simulink model "MyRhoVar"  (Simulink 7.9)
settings: Solver=FixedStepDiscrete  StartTime=0.0  StopTime=1e8  FixedStep=1  RelTol=1e-3
(part 2 of 3)

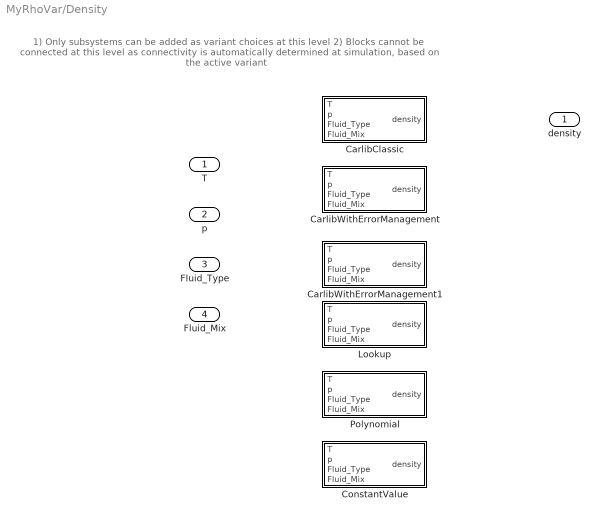
== system MyRhoVar/Density ==
  note: 1) Only subsystems can be added as variant choices at this level
      | 2) Blocks cannot be connected at this level as connectivity is
      | automatically determined at simulation, based on the active variant
  T : Inport
  p : Inport  Port=2
  Fluid_Type : Inport  Port=3
  Fluid_Mix : Inport  Port=4
  CarlibClassic : Subsystem  VariantObject=CarlibClassic  mask{INPUTARGUMENTS=INPUTARGUMENTS, DUMMY=0, ACTIVE=0, UNUSEDINPORTS=UNUSEDINPORTS}
      mask init:
      | Inports=find_system(gcb,'LookUnderMasks','all','FollowLinks','on','SearchDepth',1,'BlockType','Inport');
      | Constants=find_system(gcb,'LookUnderMasks','all','FollowLinks','on','SearchDepth',1,'BlockType','Constant');
      | Selectors=find_system(gcb,'LookUnderMasks','all','FollowLinks','on','SearchDepth',1,'BlockType','Selector');
      | BusSelectors=find_system(gcb,'LookUnderMasks','all','FollowLinks','on','SearchDepth',1,'BlockType','BusSelector');
      | Demuxes=find_system(gcb,'LookUnderMasks','all','FollowLinks','on','SearchDepth',1,'BlockType','Demux');
      | Terminators=find_system(gcb,'LookUnderMasks','all','FollowLinks','on','SearchDepth',1,'BlockType','Terminator');
      | 
      | %%delete lines, Demuxes, Selectors, Bus Selectors, Constants
      | %delete all lines
      | for Count=1:numel(Inports)
      |     AuxVar=get_param(Inports{Count},'LineHandles');
      |     for Count2=1:numel(AuxVar.Outport)
      |         if AuxVar.Outport>=0
      |             delete_line(AuxVar.Outport(Count2));
      |         end
      |     end
      | end
      | for Count=1:numel(Constants)
      |     AuxVar=get_param(Constants{Count},'LineHandles');
      |     for Count2=1:numel(AuxVar.Outport)
      |         if AuxVar.Outport>=0
      |             delete_line(AuxVar.Outport(Count2));
      |         end
      |     end
      | end
      | for Count=1:numel(Selectors)
      |     AuxVar=get_param(Selectors{Count},'LineHandles');
      |     for Count2=1:numel(AuxVar.Outport)
      |         if AuxVar.Outport>=0
      |             delete_line(AuxVar.Outport(Count2));
      |         end
      |     end
      | end
      | for Count=1:numel(BusSelectors)
      |     AuxVar=get_param(BusSelectors{Count},'LineHandles');
      |     for Count2=1:numel(AuxVar.Outport)
      |         if AuxVar.Outport>=0
      |             delete_line(AuxVar.Outport(Count2));
      |         end
      |     end
      | end
      | for Count=1:numel(Demuxes)
      |     AuxVar=get_param(Demuxes{Count},'LineHandles');
      |     for Count2=1:numel(AuxVar.Outport)
      |         if AuxVar.Outport>=0
      |             delete_line(AuxVar.Outport(Count2));
      |         end
      |     end
      | end
      | clear Count Count2 AuxVar;
      | 
      | %delete all constants, selectos, bus selectors and demuxes
      | for Count=1:numel(Constants)
      |     delete_block(Constants{Count})
      | end
      | for Count=1:numel(Selectors)
      |     delete_block(Selectors{Count})
      | end
      | for Count=1:numel(BusSelectors)
      |     delete_block(BusSelectors{Count})
      | end
      | for Count=1:numel(Demuxes)
      |     delete_block(Demuxes{Count})
      | end
      | for Count=1:numel(Terminators)
      |     delete_block(Terminators{Count})
      | end
      | clear Count;
      |     
      | 
      | %%add / delete inports and add constants and lines
      | if ACTIVE==1
      |     if INPUTARGUMENTS==1 || INPUTARGUMENTS==2 %T p ID Mix
      |         %delete all unused inports
      |         for Count=5:numel(Inports)
      |             delete_block(Inports{Count});
      |         end
      |         InportsMyParent=find_system(get_param(gcb,'Parent'),'LookUnderMasks','all','FollowLinks','on','SearchDepth',1,'BlockType','Inport');
      |         for Count=5:numel(InportsMyParent)
      |             delete_block(InportsMyParent{Count});
      |         end
      |         clear InPortsMyParent;
      |         
      |         if numel(Inports)>=1
      |             set_param(Inports{1},'Name','T');
      |         else
      |             add_block('built-in/Inport',[gcb,'/T']);
      |         end
      |         set_param([gcb,'/T'],'Position',[55   243    85   257]);
      |         add_line(gcb,'T/1','rhofluid/3');
      |         if numel(Inports)>=2
      |             set_param(Inports{2},'Name','p');
      |         else
      |             add_block('built-in/Inport',[gcb,'/p']);
      |         end
      |         set_param([gcb,'/p'],'Position',[55   313    85   327]);
      |         add_line(gcb,'p/1','rhofluid/4');
      |         if numel(Inports)>=3
      |             set_param(Inports{3},'Name','Fluid_Type');
      |         else
      |             add_block('built-in/Inport',[gcb,'/Fluid_Type']);
      |         end
      |         set_param([gcb,'/Fluid_Type'],'Position',[55   103    85   117]);
      |         add_line(gcb,'Fluid_Type/1','rhofluid/1');
      |         if numel(Inports)>=4
      |             set_param(Inports{4},'Name','Fluid_Mix');
      |         else
      |             add_block('built-in/Inport',[gcb,'/Fluid_Mix']);
      |         end
      |         set_param([gcb,'/Fluid_Mix'],'Position',[55   173    85   187]);
      |         add_line(gcb,'Fluid_Mix/1','rhofluid/2');
      |     elseif INPUTARGUMENTS==3 %THV
      |         %delete all unused inports
      |         for Count=2:numel(Inports)
      |             delete_block(Inports{Count});
      |         end
      |         InportsMyParent=find_system(get_param(gcb,'Parent'),'LookUnderMasks','all','FollowLinks','on','SearchDepth',1,'BlockType','Inport');
      |         for Count=2:numel(InportsMyParent)
      |             delete_block(InportsMyParent{Count});
      |         end
      |         clear InPortsMyParent;
      |         clear Count;
      |         
      |         if numel(Inports)>=1
      |             set_param(Inports{1},'Name','THV');
      |         else
      |             add_block('built-in/Inport',[gcb,'/THV']);
      |         end
      |         set_param([gcb,'/THV'],'Position',[55   208    85   222]);
      |         add_block('built-in/Selector',[gcb,'/Selector']); %add a selector
      |         set_param([gcb,'/Selector'],'Position',[125   196   165   234]);
      |         set_param([gcb,'/Selector'],'InputPortWidth','-1')
      |         set_param([gcb,'/Selector'],'Indices','[5 6 2 4]');
      |         add_block('built-in/Demux',[gcb,'/Demux']); %add a demux
      |         set_param([gcb,'/Demux'],'Position',[220    73   225   357]);
      |         set_param([gcb,'/Demux'],'Outputs','4');
      |         add_line(gcb,'THV/1','Selector/1');
      |         add_line(gcb,'Selector/1','Demux/1');
      |         add_line(gcb,'Demux/1','rhofluid/1');
      |         add_line(gcb,'Demux/2','rhofluid/2');
      |         add_line(gcb,'Demux/3','rhofluid/3');
      |         add_line(gcb,'Demux/4','rhofluid/4');
      |     elseif INPUTARGUMENTS==4 %THB
      |         %delete all unused inports
      |         for Count=2:numel(Inports)
      |             delete_block(Inports{Count});
      |         end
      |         InportsMyParent=find_system(get_param(gcb,'Parent'),'LookUnderMasks','all','FollowLinks','on','SearchDepth',1,'BlockType','Inport');
      |         for Count=2:numel(InportsMyParent)
      |             delete_block(InportsMyParent{Count});
      |         end
      |         clear InPortsMyParent;
      |         clear Count;
      |         
      |         if numel(Inports)>=1
      |             set_param(Inports{1},'Name','THB');
      |         else
      |             add_block('built-in/Inport',[gcb,'/THB']);
      |         end
      |         set_param([gcb,'/THB'],'Position',[55   208    85   222]);
      |         add_block('built-in/BusSelector',[gcb,'/BusSelector']); %add a bus selector
      |         set_param([gcb,'/BusSelector'],'Position',[220    73   225   357]);
      |         set_param([gcb,'/BusSelector'],'OutputSignals','FluidType,FluidMix,Temperature,Pressure');
      |         add_line(gcb,'THB/1','BusSelector/1');
      |         add_line(gcb,'BusSelector/1','rhofluid/1');
      |         add_line(gcb,'BusSelector/2','rhofluid/2');
      |         add_line(gcb,'BusSelector/3','rhofluid/3');
      |         add_line(gcb,'BusSelector/4','rhofluid/4');
      |     end
      | else
      |     for Count=numel(UNUSEDINPORTS)+1:numel(Inports) %delete all unused inports
      |         delete_block(Inports{Count});
      |     end
      |     for Count=1:numel(UNUSEDINPORTS)
      |         if numel(Inports)<Count
      |             add_block('built-in/Inport',[gcb,'/',UNUSEDINPORTS{Count}]);
      |         else
      |             set_param(Inports{Count},'Name',UNUSEDINPORTS{Count});
      |         end
      |         set_param([gcb,'/',UNUSEDINPORTS{Count}],'Position',[55 50*Count 85 50*Count+14]);
      |         add_block('built-in/Terminator',[gcb,'/Terminator_',UNUSEDINPORTS{Count}]);
      |         set_param([gcb,'/Terminator_',UNUSEDINPORTS{Count}],'Position',[155 50*Count-3 175 50*Count+17]);
      |         add_line(gcb,[UNUSEDINPORTS{Count},'/1'],['Terminator_',UNUSEDINPORTS{Count},'/1']);
      |     end
      |     add_block('built-in/Constant',[gcb,'/Constant_T']);
      |     set_param([gcb,'/Constant_T'],'Position',[275   235   305   265]);
      |     set_param([gcb,'/Constant_T'],'Value','20.0');
      |     add_line(gcb,'Constant_T/1','rhofluid/3');
      |     
      |     add_block('built-in/Constant',[gcb,'/Constant_p']);
      |     set_param([gcb,'/Constant_p'],'Position',[275   305   305   335]);
      |     set_param([gcb,'/Constant_p'],'Value','1e5');
      |     add_line(gcb,'Constant_p/1','rhofluid/4');
      |     
      |     add_block('built-in/Constant',[gcb,'/Constant_Type']);
      |     set_param([gcb,'/Constant_Type'],'Position',[275    95   305   125]);
      |     set_param([gcb,'/Constant_Type'],'Value','1');
      |     add_line(gcb,'Constant_Type/1','rhofluid/1');
      |     
      |     add_block('built-in/Constant',[gcb,'/Constant_Mix']);
      |     set_param([gcb,'/Constant_Mix'],'Position',[275   165   305   195]);
      |     set_param([gcb,'/Constant_Mix'],'Value','0.0');
      |     add_line(gcb,'Constant_Mix/1','rhofluid/2');
      | end
  CarlibWithErrorManagement : Subsystem  VariantObject=CarlibWithErrorManagement  mask{INPUTARGUMENTS=INPUTARGUMENTS, MAXTOTALWARNINGS=MAXTOTALWARNINGS, MAXCONSECUTIVEWARNINGS=MAXCONSECUTIVEWARNINGS, DUMMY=1, ACTIVE=0, UNUSEDINPORTS=UNUSEDINPORTS, DEBUGLEVEL=DEBUGLEVEL, WRITETOFILE=WRITETOFILE, FILENAME=FILENAME}
      mask init: same as MyRhoVar/Density/CarlibClassic
  CarlibWithErrorManagement1 : Subsystem  VariantObject=CarlibWithErrorManagement1  mask{INPUTARGUMENTS=INPUTARGUMENTS, MAXTOTALWARNINGS=MAXTOTALWARNINGS, MAXCONSECUTIVEWARNINGS=MAXCONSECUTIVEWARNINGS, DUMMY=1, ACTIVE=1, UNUSEDINPORTS=UNUSEDINPORTS, DEBUGLEVEL=DEBUGLEVEL, WRITETOFILE=WRITETOFILE, FILENAME=FILENAME}
      mask init: same as MyRhoVar/Density/CarlibClassic
  ConstantValue : Subsystem  VariantObject=ConstantValue  mask{INPUTARGUMENTS=INPUTARGUMENTS, CONSTANTVALUE=CONSTANTVALUE, DUMMY=1, ACTIVE=0, UNUSEDINPORTS=UNUSEDINPORTS}
      mask init:
      | Inports=find_system(gcb,'LookUnderMasks','all','FollowLinks','on','SearchDepth',1,'BlockType','Inport');
      | Constants=find_system(gcb,'LookUnderMasks','all','FollowLinks','on','SearchDepth',1,'BlockType','Constant');
      | Terminators=find_system(gcb,'LookUnderMasks','all','FollowLinks','on','SearchDepth',1,'BlockType','Terminator');
      | 
      | %%delete lines, Constants and Terminators
      | %delete all lines
      | for Count=1:numel(Inports)
      |     AuxVar=get_param(Inports{Count},'LineHandles');
      |     for Count2=1:numel(AuxVar.Outport)
      |         if AuxVar.Outport>=0
      |             delete_line(AuxVar.Outport(Count2));
      |         end
      |     end
      | end
      | for Count=1:numel(Constants)
      |     AuxVar=get_param(Constants{Count},'LineHandles');
      |     for Count2=1:numel(AuxVar.Outport)
      |         if AuxVar.Outport>=0 && ~sum(strfind(Constants{Count},'ConstantValue'))
      |             delete_line(AuxVar.Outport(Count2));
      |         end
      |     end
      | end
      | clear Count Count2 AuxVar;
      | 
      | %delete all constants and terminators
      | for Count=1:numel(Constants)
      |     if ~sum(strfind(Constants{Count},'ConstantValue'))
      |         delete_block(Constants{Count})
      |     end
      | end
      | for Count=1:numel(Terminators)
      |     delete_block(Terminators{Count})
      | end
      | clear Count;
      |     
      | %%add / delete inports and add constants and lines
      | if ACTIVE==1
      |     if INPUTARGUMENTS==1 %T p ID Mix
      |         %delete all not needed inports
      |         for Count=5:numel(Inports)
      |             delete_block(Inports{Count});
      |         end
      |         InportsMyParent=find_system(get_param(gcb,'Parent'),'LookUnderMasks','all','FollowLinks','on','SearchDepth',1,'BlockType','Inport');
      |         for Count=5:numel(InportsMyParent)
      |             delete_block(InportsMyParent{Count});
      |         end
      |         clear InPortsMyParent;
      |         clear Count;
      |         
      |         %add / rename Inports
      |         if numel(Inports)>=1
      |             set_param(Inports{1},'Name','T');
      |         else
      |             add_block('built-in/Inport',[gcb,'/T']);
      |         end
      |         set_param([gcb,'/T'],'Position',[55    50    85   64]);
      |         add_block('built-in/Terminator',[gcb,'/Terminator_T']);
      |         set_param([gcb,'/Terminator_T'],'Position',[155   47    175   67]);
      |         add_line(gcb,'T/1','Terminator_T/1');
      |         if numel(Inports)>=2
      |             set_param(Inports{2},'Name','p');
      |         else
      |             add_block('built-in/Inport',[gcb,'/p']);
      |         end
      |         set_param([gcb,'/p'],'Position',[55    100    85   114]);
      |         add_block('built-in/Terminator',[gcb,'/Terminator_p']);
      |         set_param([gcb,'/Terminator_p'],'Position',[155   97    175   117]);
      |         add_line(gcb,'p/1','Terminator_p/1');
      |         if numel(Inports)>=3
      |             set_param(Inports{3},'Name','Fluid_Type');
      |         else
      |             add_block('built-in/Inport',[gcb,'/Fluid_Type']);
      |         end
      |         set_param([gcb,'/Fluid_Type'],'Position',[55   150    85   164]);
      |         add_block('built-in/Terminator',[gcb,'/Terminator_Type']);
      |         set_param([gcb,'/Terminator_Type'],'Position',[155   147    175   167]);
      |         add_line(gcb,'Fluid_Type/1','Terminator_Type/1');
      |         if numel(Inports)>=4
      |             set_param(Inports{4},'Name','Fluid_Mix');
      |         else
      |             add_block('built-in/Inport',[gcb,'/Fluid_Mix']);
      |         end
      |         set_param([gcb,'/Fluid_Mix'],'Position',[55   200    85   214]);
      |         add_block('built-in/Terminator',[gcb,'/Terminator_Mix']);
      |         set_param([gcb,'/Terminator_Mix'],'Position',[155   197    175   217]);
      |         add_line(gcb,'Fluid_Mix/1','Terminator_Mix/1');
      |     elseif INPUTARGUMENTS==2 %no input
      |         %delete all unused inports
      |         for Count=1:numel(Inports)
      |             delete_block(Inports{Count});
      |         end
      |         InportsMyParent=find_system(get_param(gcb,'Parent'),'LookUnderMasks','all','FollowLinks','on','SearchDepth',1,'BlockType','Inport');
      |         for Count=1:numel(InportsMyParent)
      |             delete_block(InportsMyParent{Count});
      |         end
      |         clear InPortsMyParent;
      |         clear Count;
      |     elseif INPUTARGUMENTS==3 %THV
      |         %delete all unused inports
      |         for Count=2:numel(Inports)
      |             delete_block(Inports{Count});
      |         end
      |         InportsMyParent=find_system(get_param(gcb,'Parent'),'LookUnderMasks','all','FollowLinks','on','SearchDepth',1,'BlockType','Inport');
      |         for Count=2:numel(InportsMyParent)
      |             delete_block(InportsMyParent{Count});
      |         end
      |         clear InPortsMyParent;
      |         clear Count;
      |         
      |         if numel(Inports)>=1
      |             set_param(Inports{1},'Name','THV');
      |         else
      |             add_block('built-in/Inport',[gcb,'/THV']);
      |         end
      |         set_param([gcb,'/THV'],'Position',[55    50    85   64]);
      |         add_block('built-in/Terminator',[gcb,'/Terminator_THV']);
      |         set_param([gcb,'/Terminator_THV'],'Position',[155   47    175   67]);
      |         add_line(gcb,'THV/1','Terminator_THV/1');
      |     elseif INPUTARGUMENTS==4 %THB
      |         %delete all unused inports
      |         for Count=2:numel(Inports)
      |             delete_block(Inports{Count});
      |         end
      |         InportsMyParent=find_system(get_param(gcb,'Parent'),'LookUnderMasks','all','FollowLinks','on','SearchDepth',1,'BlockType','Inport');
      |         for Count=2:numel(InportsMyParent)
      |             delete_block(InportsMyParent{Count});
      |         end
      |         clear InPortsMyParent;
      |         clear Count;
      |         
      |         if numel(Inports)>=1
      |             set_param(Inports{1},'Name','THB');
      |         else
      |             add_block('built-in/Inport',[gcb,'/THB']);
      |         end
      |         set_param([gcb,'/THB'],'Position',[55    50    85   64]);
      |         add_block('built-in/Terminator',[gcb,'/Terminator_THB']);
      |         set_param([gcb,'/Terminator_THB'],'Position',[155   47    175   67]);
      |         add_line(gcb,'THB/1','Terminator_THB/1');
      |     end
      | else
      |     for Count=numel(UNUSEDINPORTS)+1:numel(Inports) %delete all unused inports
      |         delete_block(Inports{Count});
      |     end
      |     for Count=1:numel(UNUSEDINPORTS)
      |         if numel(Inports)<Count
      |             add_block('built-in/Inport',[gcb,'/',UNUSEDINPORTS{Count}]);
      |         else
      |             set_param(Inports{Count},'Name',UNUSEDINPORTS{Count});
      |         end
      |         set_param([gcb,'/',UNUSEDINPORTS{Count}],'Position',[55 50*Count 85 50*Count+14]);
      |         add_block('built-in/Terminator',[gcb,'/Terminator_',UNUSEDINPORTS{Count}]);
      |         set_param([gcb,'/Terminator_',UNUSEDINPORTS{Count}],'Position',[155 50*Count-3 175 50*Count+17]);
      |         add_line(gcb,[UNUSEDINPORTS{Count},'/1'],['Terminator_',UNUSEDINPORTS{Count},'/1']);
      |     end
      | end
  Lookup : Subsystem  VariantObject=Lookup  mask{INPUTARGUMENTS=INPUTARGUMENTS, TLOOKUP=TLOOKUP, PLOOKUP=PLOOKUP, MIXLOOKUP=MIXLOOKUP, DENSITYLOOKUP=DENSITYLOOKUP, DUMMY=1, ACTIVE=0, UNUSEDINPORTS=UNUSEDINPORTS}
      mask init:
      | Inports=find_system(gcb,'LookUnderMasks','all','FollowLinks','on','SearchDepth',1,'BlockType','Inport');
      | Constants=find_system(gcb,'LookUnderMasks','all','FollowLinks','on','SearchDepth',1,'BlockType','Constant');
      | Selectors=find_system(gcb,'LookUnderMasks','all','FollowLinks','on','SearchDepth',1,'BlockType','Selector');
      | BusSelectors=find_system(gcb,'LookUnderMasks','all','FollowLinks','on','SearchDepth',1,'BlockType','BusSelector');
      | Demuxes=find_system(gcb,'LookUnderMasks','all','FollowLinks','on','SearchDepth',1,'BlockType','Demux');
      | Terminators=find_system(gcb,'LookUnderMasks','all','FollowLinks','on','SearchDepth',1,'BlockType','Terminator');
      | 
      | %%delete lines, Demuxes, Selectors, Bus Selectors, Constants
      | %delete all lines
      | for Count=1:numel(Inports)
      |     AuxVar=get_param(Inports{Count},'LineHandles');
      |     for Count2=1:numel(AuxVar.Outport)
      |         if AuxVar.Outport>=0
      |             delete_line(AuxVar.Outport(Count2));
      |         end
      |     end
      | end
      | for Count=1:numel(Constants)
      |     AuxVar=get_param(Constants{Count},'LineHandles');
      |     for Count2=1:numel(AuxVar.Outport)
      |         if AuxVar.Outport>=0
      |             delete_line(AuxVar.Outport(Count2));
      |         end
      |     end
      | end
      | for Count=1:numel(Selectors)
      |     AuxVar=get_param(Selectors{Count},'LineHandles');
      |     for Count2=1:numel(AuxVar.Outport)
      |         if AuxVar.Outport>=0
      |             delete_line(AuxVar.Outport(Count2));
      |         end
      |     end
      | end
      | for Count=1:numel(BusSelectors)
      |     AuxVar=get_param(BusSelectors{Count},'LineHandles');
      |     for Count2=1:numel(AuxVar.Outport)
      |         if AuxVar.Outport>=0
      |             delete_line(AuxVar.Outport(Count2));
      |         end
      |     end
      | end
      | for Count=1:numel(Demuxes)
      |     AuxVar=get_param(Demuxes{Count},'LineHandles');
      |     for Count2=1:numel(AuxVar.Outport)
      |         if AuxVar.Outport>=0
      |             delete_line(AuxVar.Outport(Count2));
      |         end
      |     end
      | end
      | clear Count Count2 AuxVar;
      | 
      | %delete all constants, selectos, bus selectors and demuxes
      | for Count=1:numel(Constants)
      |     delete_block(Constants{Count})
      | end
      | for Count=1:numel(Selectors)
      |     delete_block(Selectors{Count})
      | end
      | for Count=1:numel(BusSelectors)
      |     delete_block(BusSelectors{Count})
      | end
      | for Count=1:numel(Demuxes)
      |     delete_block(Demuxes{Count})
      | end
      | for Count=1:numel(Terminators)
      |     delete_block(Terminators{Count})
      | end
      | clear Count;
      |     
      | %%add / delete inports and add constants and lines
      | if ACTIVE==1
      |     if INPUTARGUMENTS==1 %T p ID Mix
      |         %delete all not needed inports
      |         for Count=5:numel(Inports)
      |             delete_block(Inports{Count});
      |         end
      |         InportsMyParent=find_system(get_param(gcb,'Parent'),'LookUnderMasks','all','FollowLinks','on','SearchDepth',1,'BlockType','Inport');
      |         for Count=5:numel(InportsMyParent)
      |             delete_block(InportsMyParent{Count});
      |         end
      |         clear InPortsMyParent;
      |         
      |         if numel(Inports)>=1
      |             set_param(Inports{1},'Name','T');
      |         else
      |             add_block('built-in/Inport',[gcb,'/T']);
      |         end
      |         set_param([gcb,'/T'],'Position',[55    63    85    77]);
      |         add_line(gcb,'T/1','LookupTable/1');
      |         if numel(Inports)>=2
      |             set_param(Inports{2},'Name','p');
      |         else
      |             add_block('built-in/Inport',[gcb,'/p']);
      |         end
      |         set_param([gcb,'/p'],'Position',[55    93    85   107]);
      |         add_line(gcb,'p/1','LookupTable/2');
      |         if numel(Inports)>=3
      |             set_param(Inports{3},'Name','Fluid_Type');
      |         else
      |             add_block('built-in/Inport',[gcb,'/Fluid_Type']);
      |         end
      |         set_param([gcb,'/Fluid_Type'],'Position',[55   153    85   167]);
      |         add_block('built-in/Terminator',[gcb,'/Terminator_Type']);
      |         set_param([gcb,'/Terminator_Type'],'Position',[155   150    175   170]);
      |         add_line(gcb,'Fluid_Type/1','Terminator_Type/1');
      |         if numel(Inports)>=4
      |             set_param(Inports{4},'Name','Fluid_Mix');
      |         else
      |             add_block('built-in/Inport',[gcb,'/Fluid_Mix']);
      |         end
      |         set_param([gcb,'/Fluid_Mix'],'Position',[55   123    85   137]);
      |         add_line(gcb,'Fluid_Mix/1','LookupTable/3');
      |     elseif INPUTARGUMENTS==2 %T, p, Mix
      |         %delete all not needed inports
      |         for Count=4:numel(Inports)
      |             delete_block(Inports{Count});
      |         end
      |         InportsMyParent=find_system(get_param(gcb,'Parent'),'LookUnderMasks','all','FollowLinks','on','SearchDepth',1,'BlockType','Inport');
      |         for Count=4:numel(InportsMyParent)
      |             delete_block(InportsMyParent{Count});
      |         end
      |         clear InportsMyParent;
      |         
      |         %add / rename inports
      |         if numel(Inports)>=1
      |             set_param(Inports{1},'Name','T');
      |         else
      |             add_block('built-in/Inport',[gcb,'/T']);
      |         end
      |         set_param([gcb,'/T'],'Position',[55    63    85    77]);
      |         add_line(gcb,'T/1','LookupTable/1');
      |         if numel(Inports)>=2
      |             set_param(Inports{2},'Name','p');
      |         else
      |             add_block('built-in/Inport',[gcb,'/p']);
      |         end
      |         set_param([gcb,'/p'],'Position',[55    93    85   107]);
      |         add_line(gcb,'p/1','LookupTable/2');
      |         if numel(Inports)>=3
      |             set_param(Inports{3},'Name','Fluid_Mix');
      |         else
      |             add_block('built-in/Inport',[gcb,'/Fluid_Mix']);
      |         end
      |         set_param([gcb,'/Fluid_Mix'],'Position',[55   123    85   137]);
      |         add_line(gcb,'Fluid_Mix/1','LookupTable/3');
      |     elseif INPUTARGUMENTS==3 %THV
      |         for Count=2:numel(Inports) %delete all but the first inport
      |             delete_block(Inports{Count});
      |         end
      |         InportsMyParent=find_system(get_param(gcb,'Parent'),'LookUnderMasks','all','FollowLinks','on','SearchDepth',1,'BlockType','Inport');
      |         for Count=2:numel(InportsMyParent)
      |             delete_block(InportsMyParent{Count});
      |         end
      |         clear InportsMyParent;
      |         clear Count;
      |         
      |         if numel(Inports)>=1
      |             set_param(Inports{1},'Name','THV');
      |         else
      |             add_block('built-in/Inport',[gcb,'/THV']);
      |         end
      |         set_param([gcb,'/THV'],'Position',[55    93    85   107]);
      |         add_block('built-in/Selector',[gcb,'/Selector']); %add a selector
      |         set_param([gcb,'/Selector'],'Position',[125    81   165   119]);
      |         set_param([gcb,'/Selector'],'InputPortWidth','-1')
      |         set_param([gcb,'/Selector'],'Indices','[2 4 6]');
      |         add_block('built-in/Demux',[gcb,'/Demux']); %add a demux
      |         set_param([gcb,'/Demux'],'Position',[220    52   225   148]);
      |         set_param([gcb,'/Demux'],'Outputs','3');
      |         add_line(gcb,'THV/1','Selector/1');
      |         add_line(gcb,'Selector/1','Demux/1');
      |         add_line(gcb,'Demux/1','LookupTable/1');
      |         add_line(gcb,'Demux/2','LookupTable/2');
      |         add_line(gcb,'Demux/3','LookupTable/3');
      |     elseif INPUTARGUMENTS==4 %THB
      |         for Count=2:numel(Inports) %delete all but the first inport
      |             delete_block(Inports{Count});
      |         end
      |         InportsMyParent=find_system(get_param(gcb,'Parent'),'LookUnderMasks','all','FollowLinks','on','SearchDepth',1,'BlockType','Inport');
      |         for Count=2:numel(InportsMyParent)
      |             delete_block(InportsMyParent{Count});
      |         end
      |         clear InportsMyParent;
      |         clear Count;
      |         
      |         if numel(Inports)>=1
      |             set_param(Inports{1},'Name','THB');
      |         else
      |             add_block('built-in/Inport',[gcb,'/THB']);
      |         end
      |         set_param([gcb,'/THB'],'Position',[55    93    85   107]);
      |         add_block('built-in/BusSelector',[gcb,'/BusSelector']); %add a bus selector
      |         set_param([gcb,'/BusSelector'],'Position',[220    53   225   147]);
      |         set_param([gcb,'/BusSelector'],'OutputSignals','Temperature,Pressure,FluidMix');
      |         add_line(gcb,'THB/1','BusSelector/1');
      |         add_line(gcb,'BusSelector/1','LookupTable/1');
      |         add_line(gcb,'BusSelector/2','LookupTable/2');
      |         add_line(gcb,'BusSelector/3','LookupTable/3');
      |     end
      | else
      |     %delete all unused inports
      |     for Count=numel(UNUSEDINPORTS)+1:numel(Inports)
      |         delete_block(Inports{Count});
      |     end
      |     
      |     for Count=1:numel(UNUSEDINPORTS)
      |         if numel(Inports)<Count
      |             add_block('built-in/Inport',[gcb,'/',UNUSEDINPORTS{Count}]);
      |         else
      |             set_param(Inports{Count},'Name',UNUSEDINPORTS{Count});
      |         end
      |         set_param([gcb,'/',UNUSEDINPORTS{Count}],'Position',[55 50*Count 85 50*Count+14]);
      |         add_block('built-in/Terminator',[gcb,'/Terminator_',UNUSEDINPORTS{Count}]);
      |         set_param([gcb,'/Terminator_',UNUSEDINPORTS{Count}],'Position',[155 50*Count-3 175 50*Count+17]);
      |         add_line(gcb,[UNUSEDINPORTS{Count},'/1'],['Terminator_',UNUSEDINPORTS{Count},'/1']);
      |     end
      |     add_block('built-in/Constant',[gcb,'/Constant_T']);
      |     set_param([gcb,'/Constant_T'],'Position',[260    35   290    65]);
      |     set_param([gcb,'/Constant_T'],'Value','20.0');
      |     add_line(gcb,'Constant_T/1','LookupTable/1');
      |     
      |     add_block('built-in/Constant',[gcb,'/Constant_p']);
      |     set_param([gcb,'/Constant_p'],'Position',[260    85   290    115]);
      |     set_param([gcb,'/Constant_p'],'Value','1e5');
      |     add_line(gcb,'Constant_p/1','LookupTable/2');
      |     
      |     add_block('built-in/Constant',[gcb,'/Constant_Mix']);
      |     set_param([gcb,'/Constant_Mix'],'Position',[260    135   290    165]);
      |     set_param([gcb,'/Constant_Mix'],'Value','0.0');
      |     add_line(gcb,'Constant_Mix/1','LookupTable/3');
      | end
  Polynomial : Subsystem  VariantObject=Polynomial  mask{INPUTARGUMENTS=INPUTARGUMENTS, POLYNOMIALCOEFFICIENTS=POLYNOMIALCOEFFICIENTS, DUMMY=1, ACTIVE=0, UNUSEDINPORTS=UNUSEDINPORTS}
      mask init:
      | Inports=find_system(gcb,'LookUnderMasks','all','FollowLinks','on','SearchDepth',1,'BlockType','Inport');
      | Constants=find_system(gcb,'LookUnderMasks','all','FollowLinks','on','SearchDepth',1,'BlockType','Constant');
      | Selectors=find_system(gcb,'LookUnderMasks','all','FollowLinks','on','SearchDepth',1,'BlockType','Selector');
      | BusSelectors=find_system(gcb,'LookUnderMasks','all','FollowLinks','on','SearchDepth',1,'BlockType','BusSelector');
      | Terminators=find_system(gcb,'LookUnderMasks','all','FollowLinks','on','SearchDepth',1,'BlockType','Terminator');
      | 
      | %%delete lines, Demuxes, Selectors, Bus Selectors, Constants and
      | %%Terminators
      | %delete all lines
      | for Count=1:numel(Inports)
      |     AuxVar=get_param(Inports{Count},'LineHandles');
      |     for Count2=1:numel(AuxVar.Outport)
      |         if AuxVar.Outport>=0
      |             delete_line(AuxVar.Outport(Count2));
      |         end
      |     end
      | end
      | for Count=1:numel(Constants)
      |     AuxVar=get_param(Constants{Count},'LineHandles');
      |     for Count2=1:numel(AuxVar.Outport)
      |         if AuxVar.Outport>=0
      |             delete_line(AuxVar.Outport(Count2));
      |         end
      |     end
      | end
      | for Count=1:numel(Selectors)
      |     AuxVar=get_param(Selectors{Count},'LineHandles');
      |     for Count2=1:numel(AuxVar.Outport)
      |         if AuxVar.Outport>=0
      |             delete_line(AuxVar.Outport(Count2));
      |         end
      |     end
      | end
      | for Count=1:numel(BusSelectors)
      |     AuxVar=get_param(BusSelectors{Count},'LineHandles');
      |     for Count2=1:numel(AuxVar.Outport)
      |         if AuxVar.Outport>=0
      |             delete_line(AuxVar.Outport(Count2));
      |         end
      |     end
      | end
      | clear Count Count2 AuxVar;
      | 
      | %delete all constants, selectos, bus selectors and terminators
      | for Count=1:numel(Constants)
      |     delete_block(Constants{Count})
      | end
      | for Count=1:numel(Selectors)
      |     delete_block(Selectors{Count})
      | end
      | for Count=1:numel(BusSelectors)
      |     delete_block(BusSelectors{Count})
      | end
      | for Count=1:numel(Terminators)
      |     delete_block(Terminators{Count})
      | end
      | clear Count;
      |     
      | %%add / delete inports and add constants and lines
      | if ACTIVE==1
      |     if INPUTARGUMENTS==1 %T p ID Mix
      |         %delete all not needed inports
      |         for Count=5:numel(Inports)
      |             delete_block(Inports{Count});
      |         end
      |         InportsMyParent=find_system(get_param(gcb,'Parent'),'LookUnderMasks','all','FollowLinks','on','SearchDepth',1,'BlockType','Inport');
      |         for Count=5:numel(InportsMyParent)
      |             delete_block(InportsMyParent{Count});
      |         end
      |         clear InPortsMyParent;
      |         clear Count;
      |         
      |         %add / rename Inports
      |         if numel(Inports)>=1
      |             set_param(Inports{1},'Name','T');
      |         else
      |             add_block('built-in/Inport',[gcb,'/T']);
      |         end
      |         set_param([gcb,'/T'],'Position',[55    50    85   64]);
      |         add_line(gcb,'T/1','Polynomial/1');
      |         if numel(Inports)>=2
      |             set_param(Inports{2},'Name','p');
      |         else
      |             add_block('built-in/Inport',[gcb,'/p']);
      |         end
      |         set_param([gcb,'/p'],'Position',[55    100    85   114]);
      |         add_block('built-in/Terminator',[gcb,'/Terminator_p']);
      |         set_param([gcb,'/Terminator_p'],'Position',[155   97    175   117]);
      |         add_line(gcb,'p/1','Terminator_p/1');
      |         if numel(Inports)>=3
      |             set_param(Inports{3},'Name','Fluid_Type');
      |         else
      |             add_block('built-in/Inport',[gcb,'/Fluid_Type']);
      |         end
      |         set_param([gcb,'/Fluid_Type'],'Position',[55   150    85   164]);
      |         add_block('built-in/Terminator',[gcb,'/Terminator_Type']);
      |         set_param([gcb,'/Terminator_Type'],'Position',[155   147    175   167]);
      |         add_line(gcb,'Fluid_Type/1','Terminator_Type/1');
      |         if numel(Inports)>=4
      |             set_param(Inports{4},'Name','Fluid_Mix');
      |         else
      |             add_block('built-in/Inport',[gcb,'/Fluid_Mix']);
      |         end
      |         set_param([gcb,'/Fluid_Mix'],'Position',[55   200    85   214]);
      |         add_block('built-in/Terminator',[gcb,'/Terminator_Mix']);
      |         set_param([gcb,'/Terminator_Mix'],'Position',[155   197    175   217]);
      |         add_line(gcb,'Fluid_Mix/1','Terminator_Mix/1');
      |     elseif INPUTARGUMENTS==2 %T
      |         %delete all unused inports
      |         for Count=2:numel(Inports)
      |             delete_block(Inports{Count});
      |         end
      |         InportsMyParent=find_system(get_param(gcb,'Parent'),'LookUnderMasks','all','FollowLinks','on','SearchDepth',1,'BlockType','Inport');
      |         for Count=2:numel(InportsMyParent)
      |             delete_block(InportsMyParent{Count});
      |         end
      |         clear InPortsMyParent;
      |         clear Count;
      |         
      |         if numel(Inports)>=1
      |             set_param(Inports{1},'Name','T');
      |         else
      |             add_block('built-in/Inport',[gcb,'/T']);
      |         end
      |         set_param([gcb,'/T'],'Position',[55    50    85   64]);
      |         add_line(gcb,'T/1','Polynomial/1');
      |     elseif INPUTARGUMENTS==3 %THV
      |         %delete all unused inports
      |         for Count=2:numel(Inports)
      |             delete_block(Inports{Count});
      |         end
      |         InportsMyParent=find_system(get_param(gcb,'Parent'),'LookUnderMasks','all','FollowLinks','on','SearchDepth',1,'BlockType','Inport');
      |         for Count=2:numel(InportsMyParent)
      |             delete_block(InportsMyParent{Count});
      |         end
      |         clear InPortsMyParent;
      |         clear Count;
      |         
      |         if numel(Inports)>=1
      |             set_param(Inports{1},'Name','THV');
      |         else
      |             add_block('built-in/Inport',[gcb,'/THV']);
      |         end
      |         set_param([gcb,'/THV'],'Position',[55    50    85   64]);
      |         add_block('built-in/Selector',[gcb,'/Selector']); %add a selector
      |         set_param([gcb,'/Selector'],'Position',[125    36   165    74]);
      |         set_param([gcb,'/Selector'],'InputPortWidth','-1')
      |         set_param([gcb,'/Selector'],'Indices','[2]');
      |         add_line(gcb,'THV/1','Selector/1');
      |         add_line(gcb,'Selector/1','Polynomial/1');
      |     elseif INPUTARGUMENTS==4 %THB
      |         %delete all unused inports
      |         for Count=2:numel(Inports)
      |             delete_block(Inports{Count});
      |         end
      |         InportsMyParent=find_system(get_param(gcb,'Parent'),'LookUnderMasks','all','FollowLinks','on','SearchDepth',1,'BlockType','Inport');
      |         for Count=2:numel(InportsMyParent)
      |             delete_block(InportsMyParent{Count});
      |         end
      |         clear InPortsMyParent;
      |         clear Count;
      |         
      |         if numel(Inports)>=1
      |             set_param(Inports{1},'Name','THB');
      |         else
      |             add_block('built-in/Inport',[gcb,'/THB']);
      |         end
      |         set_param([gcb,'/THB'],'Position',[55    50    85   64]);
      |         add_block('built-in/BusSelector',[gcb,'/BusSelector']); %add a bus selector
      |         set_param([gcb,'/BusSelector'],'Position',[220    36   225    74]);
      |         set_param([gcb,'/BusSelector'],'OutputSignals','Temperature');
      |         add_line(gcb,'THB/1','BusSelector/1');
      |         add_line(gcb,'BusSelector/1','Polynomial/1');
      |     end
      | else
      |     for Count=numel(UNUSEDINPORTS)+1:numel(Inports) %delete all unused inports
      |         delete_block(Inports{Count});
      |     end
      |     for Count=1:numel(UNUSEDINPORTS)
      |         if numel(Inports)<Count
      |             add_block('built-in/Inport',[gcb,'/',UNUSEDINPORTS{Count}]);
      |         else
      |             set_param(Inports{Count},'Name',UNUSEDINPORTS{Count});
      |         end
      |         set_param([gcb,'/',UNUSEDINPORTS{Count}],'Position',[55 50*Count 85 50*Count+14]);
      |         add_block('built-in/Terminator',[gcb,'/Terminator_',UNUSEDINPORTS{Count}]);
      |         set_param([gcb,'/Terminator_',UNUSEDINPORTS{Count}],'Position',[155 50*Count-3 175 50*Count+17]);
      |         add_line(gcb,[UNUSEDINPORTS{Count},'/1'],['Terminator_',UNUSEDINPORTS{Count},'/1']);
      |     end
      |     add_block('built-in/Constant',[gcb,'/Constant_T']);
      |     set_param([gcb,'/Constant_T'],'Position',[230    40   260    70]);
      |     set_param([gcb,'/Constant_T'],'Value','20.0');
      |     add_line(gcb,'Constant_T/1','Polynomial/1');
      | end
  density : Outport
